simulink model "modelnonl"  (R2016a)
settings: Solver=VariableStepAuto  StartTime=0.0  StopTime=30.0  RelTol=1e-7
values from neighbouring files (symbols this model uses):
  K = place(As,Bs,[-1 -2 -3 -4 -5 -6])    [Modelscript.m]
settings Model: Creator=Lehelxp  LastModifiedBy=Lehelxp

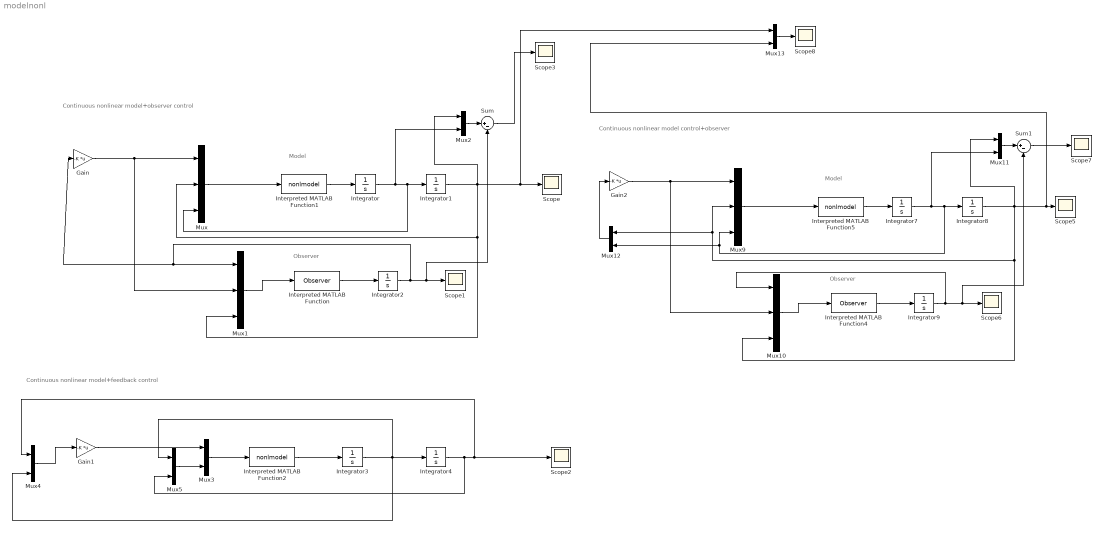
== system modelnonl ==
  note: Continuous nonlinear model+feedback control
  note: Observer
  note: Model
  note: Continuous nonlinear model+observer control
  note: Observer
  note: Model
  note: Continuous nonlinear model control+observer
  Gain : Gain  Gain=-K  Multiplication=Matrix(K*u) (u vector)
  Gain1 : Gain  Gain=-K  Multiplication=Matrix(K*u) (u vector)
  Gain2 : Gain  Gain=-K  Multiplication=Matrix(K*u) (u vector)
  Integrator : Integrator  InitialCondition=[0 0 0]'  ContinuousStateAttributes='speed'
  Integrator1 : Integrator  InitialCondition=[1 1 1]'  ContinuousStateAttributes='position'
  Integrator2 : Integrator  InitialCondition=[1 0.5 0 0 0 0]'  ContinuousStateAttributes='state.approx'
  Integrator3 : Integrator  InitialCondition=[0 0 0]'  ContinuousStateAttributes='speed'
  Integrator4 : Integrator  InitialCondition=[1 1 1]'  ContinuousStateAttributes='position'
  Integrator7 : Integrator  InitialCondition=[0 0 0]'  ContinuousStateAttributes='speed'
  Integrator8 : Integrator  InitialCondition=[1 1 1]'  ContinuousStateAttributes='position'
  Integrator9 : Integrator  InitialCondition=[1 0.5 0 0 0 0]'  ContinuousStateAttributes='state.approx'
  Interpreted MATLAB Function : MATLABFcn  MATLABFcn=Observer  OutputDimensions=6
  Interpreted MATLAB Function1 : MATLABFcn  MATLABFcn=nonlmodel  OutputDimensions=3  Output1D=off
  Interpreted MATLAB Function2 : MATLABFcn  MATLABFcn=nonlmodel  OutputDimensions=3  Output1D=off
  Interpreted MATLAB Function4 : MATLABFcn  MATLABFcn=Observer  OutputDimensions=6
  Interpreted MATLAB Function5 : MATLABFcn  MATLABFcn=nonlmodel  OutputDimensions=3  Output1D=off
  Mux{,1,9..10} (4 alike) : Mux  Inputs=3
  Mux{2..5,11..13} (7 alike) : Mux  Inputs=2
  Scope{,1..3,5..8} (8 alike) : Scope
  Sum : Sum  Inputs=|+-
  Sum1 : Sum  Inputs=|+-
  wires:
  Interpreted MATLAB Function1/1 -> Integrator/1
  Integrator/1 -> Integrator1/1, Mux/3, Mux2/2
  Integrator1/1 -> Mux13/1, Scope/1, Mux/2, Mux1/3, Mux2/1
  Mux/1 -> Interpreted MATLAB Function1/1
  Gain/1 -> Mux/1, Mux1/2
  Integrator2/1 -> Sum/2, Scope1/1, Gain/1, Mux1/1
  Mux1/1 -> Interpreted MATLAB Function/1
  Interpreted MATLAB Function/1 -> Integrator2/1
  Sum/1 -> Scope3/1
  Mux2/1 -> Sum/1
  Interpreted MATLAB Function2/1 -> Integrator3/1
  Integrator3/1 -> Mux4/2, Mux5/1, Integrator4/1
  Mux3/1 -> Interpreted MATLAB Function2/1
  Integrator4/1 -> Mux5/2, Mux4/1, Scope2/1
  Gain1/1 -> Mux3/1
  Mux4/1 -> Gain1/1
  Mux5/1 -> Mux3/2
  Interpreted MATLAB Function5/1 -> Integrator7/1
  Integrator7/1 -> Integrator8/1, Mux9/3, Mux12/2, Mux11/2
  Integrator8/1 -> Mux13/2, Scope5/1, Mux9/2, Mux12/1, Mux10/3, Mux11/1
  Mux9/1 -> Interpreted MATLAB Function5/1
  Gain2/1 -> Mux9/1, Mux10/2
  Integrator9/1 -> Mux10/1, Sum1/2, Scope6/1
  Mux10/1 -> Interpreted MATLAB Function4/1
  Interpreted MATLAB Function4/1 -> Integrator9/1
  Sum1/1 -> Scope7/1
  Mux11/1 -> Sum1/1
  Mux12/1 -> Gain2/1
  Mux13/1 -> Scope8/1
